simulink subsystem "Modelo_Piero"  (R2023b)
settings: Solver=VariableStepAuto  StartTime=0.0  StopTime=10.0  RelTol=1e-3
settings Model: Creator=Usuario_UMA  LastModifiedBy=Manuel

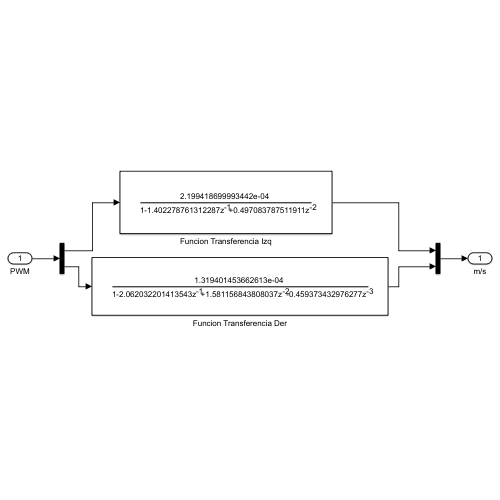
[thumbnail: Simulink's stored preview of the top-level diagram]
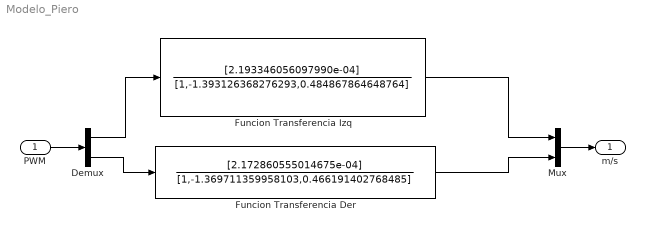
== system Modelo_Piero ==
  PWM : Inport
  Demux : Demux  Outputs=2
  Funcion Transferencia Der : DiscreteFilter  Numerator=[2.172860555014675e-04]  Denominator=[1,-1.369711359958103,0.466191402768485]
  Funcion Transferencia Izq : DiscreteFilter  Numerator=[2.193346056097990e-04]  Denominator=[1,-1.393126368276293,0.484867864648764]
  Mux : Mux  Inputs=2
  m/s : Outport
  wires:
  Mux/1 -> m/s/1
  PWM/1 -> Demux/1
  Demux/1 -> Funcion Transferencia Izq/1
  Funcion Transferencia Izq/1 -> Mux/1
  Demux/2 -> Funcion Transferencia Der/1
  Funcion Transferencia Der/1 -> Mux/2
